simulink model "final_integration"  (R2019b)
settings: Solver=FixedStepDiscrete  StartTime=0.0  StopTime=100  FixedStep=0.1  RelTol=1e-3
undefined symbols (not defined in the file): DiscIntNeverNeededParam, gcbh, rmidispblock, sigbuilder_block
libraries: simulink x2
(part 2 of 2)

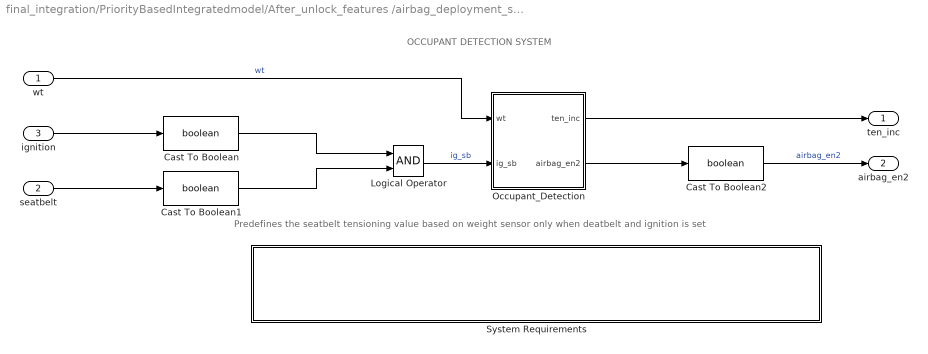
== system final_integration/PriorityBasedIntegratedmodel/After_unlock_features /airbag_deployment_system_main/occuption_detection_system ==
  note: Predefines the seatbelt tensioning value based on weight sensor only when deatbelt and ignition is set
  note: OCCUPANT DETECTION SYSTEM
  wt : Inport
  seatbelt : Inport  Port=2
  ignition : Inport  Port=3
  Cast To Boolean : DataTypeConversion  OutDataTypeStr=boolean
  Cast To Boolean1 : DataTypeConversion  OutDataTypeStr=boolean
  Cast To Boolean2 : DataTypeConversion  OutDataTypeStr=boolean
  Logical Operator : Logic  AllPortsSameDT=off  OutDataTypeStr=boolean
  Occupant_Detection : Stateflow chart  TreatAsAtomicUnit=on
  System Requirements : Subsystem  LoadFcn=rmidispblock('load',gcbh)  mask(System Requirements){id=SystemReq, title=System Requirements}
      mask prompts: title "Block Title"
      mask help: Lists the requirements for the current model.
      mask init:
      | id = 'SystemReq';
      | [w,h] = rmidispblock('display',gcbh);
      settings: CopyFcn=rmidispblock('create',gcbh)  DeleteFcn=rmidispblock('delete',gcbh)  ModelCloseFcn=rmidispblock('close',gcbh)  PreSaveFcn=rmidispblock('close',gcbh)  PostSaveFcn=rmidispblock('open',gcbh)  OpenFcn=rmidispblock('open',gcbh)  MoveFcn=rmidispblock('move',gcbh)
      mask Help: helpview(fullfile(docroot,'slrequirements','helptargets.map'),'systemrequirements')
      mask Display: text(566/2,73-4,rmidispblock('title',gcbh),'horizontalAlignment','center','verticalAlignment','top')
  ten_inc : Outport
  airbag_en2 : Outport  Port=2
  wires:
  Logical Operator/1 -> Occupant_Detection/2(ig_sb)  "ig_sb"
  Cast To Boolean1/1 -> Logical Operator/2
  Cast To Boolean/1 -> Logical Operator/1
  Occupant_Detection/1(ten_inc) -> ten_inc/1
  ignition/1 -> Cast To Boolean/1
  seatbelt/1 -> Cast To Boolean1/1
  Occupant_Detection/2(airbag_en2) -> Cast To Boolean2/1
  Cast To Boolean2/1 -> airbag_en2/1  "airbag_en2"
  wt/1 -> Occupant_Detection/1(wt)  "wt"

== system final_integration/PriorityBasedIntegratedmodel/After_unlock_features /seatbelt_warning_system/System Requirements ==
  Subsystem : Subsystem  mask{label=0, index=1}
      mask init:
      | label = rmidispblock('label',index);
      settings: OpenFcn=rmidispblock('openReq',gcbh);
      mask Display: text(0,0,label,'horizontalAlignment','left','verticalAlignment','bottom')

== system final_integration/PriorityBasedIntegratedmodel/After_unlock_features /suspension_system/System Requirements ==
  Subsystem : Subsystem  mask{label=0, index=1}
      mask init:
      | label = rmidispblock('label',index);
      settings: OpenFcn=rmidispblock('openReq',gcbh);
      mask Display: text(0,0,label,'horizontalAlignment','left','verticalAlignment','bottom')

== system final_integration/PriorityBasedIntegratedmodel/Passive Keyless Entry system/System Requirements/Subsystem ==

== system final_integration/PriorityBasedIntegratedmodel/After_unlock_features /airbag_deployment_system_main/Safe_distance_enable/System Requirements ==
  Subsystem : Subsystem  mask{label=0, index=1}
      mask init:
      | label = rmidispblock('label',index);
      settings: OpenFcn=rmidispblock('openReq',gcbh);
      mask Display: text(0,0,label,'horizontalAlignment','left','verticalAlignment','bottom')

== system final_integration/PriorityBasedIntegratedmodel/After_unlock_features /airbag_deployment_system_main/System Requirements/Subsystem ==

== system final_integration/PriorityBasedIntegratedmodel/After_unlock_features /airbag_deployment_system_main/airbag_decisionsystem/System Requirements ==
  Subsystem : Subsystem  mask{label=0, index=1}
      mask init:
      | label = rmidispblock('label',index);
      settings: OpenFcn=rmidispblock('openReq',gcbh);
      mask Display: text(0,0,label,'horizontalAlignment','left','verticalAlignment','bottom')

== system final_integration/PriorityBasedIntegratedmodel/After_unlock_features /airbag_deployment_system_main/occuption_detection_system/System Requirements ==
  Subsystem : Subsystem  mask{label=0, index=1}
      mask init:
      | label = rmidispblock('label',index);
      settings: OpenFcn=rmidispblock('openReq',gcbh);
      mask Display: text(0,0,label,'horizontalAlignment','left','verticalAlignment','bottom')

== system final_integration/PriorityBasedIntegratedmodel/After_unlock_features /seatbelt_warning_system/System Requirements/Subsystem ==

== system final_integration/PriorityBasedIntegratedmodel/After_unlock_features /suspension_system/System Requirements/Subsystem ==

== system final_integration/PriorityBasedIntegratedmodel/After_unlock_features /airbag_deployment_system_main/Safe_distance_enable/System Requirements/Subsystem ==

== system final_integration/PriorityBasedIntegratedmodel/After_unlock_features /airbag_deployment_system_main/airbag_decisionsystem/System Requirements/Subsystem ==

== system final_integration/PriorityBasedIntegratedmodel/After_unlock_features /airbag_deployment_system_main/occuption_detection_system/System Requirements/Subsystem ==

== stateflow chart final_integration/PriorityBasedIntegratedmodel/After_unlock_features /airbag_deployment_system_main/airbag_decisionsystem/Airbag_Decision ==
  state normalState
    en, du:
    airbagDeploy=0;
    seatTensioner=0;
  state standbyState
    en, du:
    airbagDeploy=0;
    seatTensioner=1;
  state fireState
    en, du:
    airbagDeploy=1;
    seatTensioner=1;
  note: 1) When no Crash(NormalState):Airbag and seatbelt tensioner are not set.
      | 2) When a crash of low or medium level(StandbyState):Seatbelt is tensioned but airbag deployment and steering retraction doesn’t take place.
      | 3) When a crash of high level(StandbyState):Seatbelt is tensioned and airbag deployment and steering retraction is also activated.
  (default) -> normalState
  standbyState -> fireState [order 1] : [vehicle_speed>=22.54]
  normalState -> standbyState : [vehicle_vol>=Vth]
  standbyState -> fireState [order 3] : [12.88<vehicle_speed<22.54]
  fireState -> standbyState : [vehicle_speed<12.88]
  standbyState -> normalState [order 2] : [vehicle_vol<Vth]
  data: Vth local =1; vehicle_speed input; vehicle_vol input; airbagDeploy output; seatTensioner output

== stateflow chart final_integration/PriorityBasedIntegratedmodel/After_unlock_features /airbag_deployment_system_main/occuption_detection_system/Occupant_Detection ==
  state systemOn
    exit:
    airbag_en2=1;
    (default) -> (junction 15) : % tension adjuster
    (junction 15) -> (junction 16) [order 1] : [wt>=75.0 && wt<=100.0]
    (junction 15) -> (junction 17) [order 2]
    (junction 16) -> (junction 24) : {ten_inc=10.0+Tini;}
    (junction 17) -> (junction 18) [order 1] : [wt>=50.0 && wt<=75.0]
    (junction 17) -> (junction 19) [order 2]
    (junction 18) -> (junction 23) : {ten_inc=20.0+Tini;}
    (junction 19) -> (junction 20) [order 1] : [wt>=25.0 && wt<=50.0]
    (junction 19) -> (junction 21) [order 2] : {ten_inc=Tini;}
    (junction 20) -> (junction 22) : {ten_inc=30.0+Tini;}
    (junction 22) -> (junction 21)
    (junction 23) -> (junction 22)
    (junction 24) -> (junction 23)
    (junction 21) -> (junction 25)
  state systemOff
    exit:
    airbag_en2=0;
  note: 1) Ignition and seatbelt is ON,then in order to avoid harsh tensioning of seat belt we read the weight sensor and accordingly set the tensioning percent.
      | 2) Ignition and Seatbelt is OFF,no seatbelt tensioning predefining takes place.
  (default) -> systemOn
  systemOn -> systemOff : [ig_sb==1.0]
  systemOff -> systemOn : [ig_sb==0]
  data: wt input; Tini local =5; ten_inc output; ig_sb input; airbag_en2 output

== stateflow chart final_integration/PriorityBasedIntegratedmodel/After_unlock_features /seatbelt_warning_system/seat_belt_alert_system ==
  state Idle_state
    en:
    seatoccupiedout=0;
    buzzer=0;
    seatbeltout=0;
  note: Input should be either 0 or 1 only
      |
      | There are 4 states:
      | Idle state: Idle means, engine is off, so there is no output
      | Seatoccupied: When passesnger enters the vehicle this state activates and the passenger seated status will be displayed on screen
      | SeatbeltOn: When seat is occupied and the passenger wears seat belt, then this state activates and the seat belt used status will be displayed
      | Buzzer: When seat is occupied nut the belt is not used, buzzer state activates and belt reminder is desplayed on screen
  state Seatoccupied
    en:
    seatoccupiedout=1;
  state Buzzer
    en:
    seatbeltout=0;
    buzzer=1;
    disp('buzzer on');
  state SeatbeltOn
    en:
    seatbeltout=1;
    buzzer=0;
  (default) -> Idle_state
  Idle_state -> Seatoccupied : [seatoccupied==1]
  SeatbeltOn -> Idle_state : [seatoccupied==0]
  Buzzer -> Idle_state [order 1] : [seatoccupied==0]
  Seatoccupied -> Buzzer [order 2] : [seatbelt==0]
  Buzzer -> SeatbeltOn [order 2] : [seatbelt==1]
  Seatoccupied -> SeatbeltOn [order 1] : [seatbelt==1]
  data: seatoccupied input; seatbelt input; seatoccupiedout output; seatbeltout output; buzzer output; c local

== stateflow chart final_integration/PriorityBasedIntegratedmodel/Passive Keyless Entry system/Door_Status_Scenario1 ==
  note: Scenario 1: When user is moving away from the source
  state PassiveENtryScenario1 [group]
    state ScanOff
    state Available
      state Signal
      state SensorWork
        state DoorSensor
          en:
          DoorEntryStatus_S1=0;
          proximity = 100;
          count=0;
          du:
          count = count +1;
          ex:
          count = 101;
        state VehicleSensor
          en:
          DoorEntryStatus_S1=0;
          proximity=750;
          count=101;
          du:
          count=count +1;
          ex:
          count = 751;
        state OutofRange
          en:
          DoorEntryStatus_S1=1;
          disp('Door is Locked');
          disp('--------------------');
          proximity=900;
          count=751;
          du:
          count=count+1;
          ex:
          count = 901;
        (default) -> DoorSensor
        DoorSensor -> VehicleSensor : [count > proximity] {disp('User moving out of Door Proximity');}
        VehicleSensor -> OutofRange : [count > proximity] {disp('User moving out of Vehicle Proximity');
            |                              disp('---------------------------------------');}
      (default) -> Signal
      SensorWork -> Signal : [Input_signal_S1==900]
      Signal -> SensorWork : [Input_signal_S1>0]{disp('Connection of the signal');
          | disp('---------------------------------------');}
    (default) -> ScanOff : {disp('---------------------------------------');
        | disp('User moving away from vehicle');
        | disp('Scanning for Signal Avalabiltiy');
        | disp('----------------------------------------');}
    Available -> ScanOff : [SignalScanInput==0]
    ScanOff -> Available : [SignalScanInput==1]{disp('Signal Available');
        | disp('---------------------------------------');}
  note: %% Vehicle Sensor
      | % When the signal value goes from 100 to 750, the Vehicle state activates
      | % When it reaches the 750 count, the door locks
  note: %% Door Sensor
      | % When the signal value goes from 0 to 100, the Door state activates
      | % When it reaches the 100 count, the still stays the same
  note: %% Door Status
      | % When both the states are active, only then the output status is given.
      | % Otherwise the door remains open
  data: proximity local; count local; Input_signal_S1 input; DoorEntryStatus_S1 output; SignalScanInput input

== stateflow chart final_integration/PriorityBasedIntegratedmodel/Passive Keyless Entry system/Door_Status_Scenario2 ==
  note: Scenario 2: When user is moving towards source
  state PassiveEntryScenario2 [group]
    state ScanOff
    state Available
      state Signal
      state SensorWork
        state OutofRange
          entry:
          DoorEntryStatus_S2=1;
          proximity = 900;
          count=899;
          during:
          count = count -1;
          exit:
          count = 749;
        state VehicleSensor
          entry:
          DoorEntryStatus_S2=1;
          proximity=750;
          count=749;
          during:
          count=count -1;
          exit:
          count = 99;
        state DoorSensor
          entry:
          DoorEntryStatus_S2=0;
          disp('Door is Unocked');
          disp('Ignition sequence allowed');
          disp('-----------------------------------');
          proximity=100;
          count=99;
          during:
          count=count - 1;
          exit:
          count = 1;
        (default) -> OutofRange
        OutofRange -> VehicleSensor : [count==749] {disp('User moving towards Vehicle Proximity');}
        VehicleSensor -> DoorSensor : [count==99] {disp('User moving towards Door Proximity');
            |                      disp('---------------------------------------');}
      (default) -> Signal
      SensorWork -> Signal : [Input_Signal_S2==0]
      Signal -> SensorWork : [Input_Signal_S2 < 1000] {disp('Connection of the signal');
          |                                          disp('---------------------------------------');}
    (default) -> ScanOff : {disp('---------------------------------------');
        | disp('User moving towards the vehicle');
        | disp('Scanning for Signal Avalabiltiy');
        | disp('----------------------------------------');}
    Available -> ScanOff : [SignalScanInput==0]
    ScanOff -> Available : [SignalScanInput==1]{disp('Signal Available');
        | disp('---------------------------------------');}
  note: %% Door Sensor
      | % When the signal value goes from 100 to 0, the Door state activates
      | % When it reaches the 0 count, the door unlocks
  note: %% Vehicle Sensor
      | % When the signal value goes from 750 to 100, the Vehicle state activates
      | % When it reaches the 100 count, the door locks
  note: %% Door Status
      | % When both the states are active, only then the output status is given.
      | % Otherwise the door remains closed
  data: proximity local; count local; Input_Signal_S2 input; DoorEntryStatus_S2 output; SignalScanInput input

== stateflow chart final_integration/PriorityBasedIntegratedmodel/After_unlock_features /suspension_system/tyremonitoring ==
  state Ignition_OFF
    en:
    F_o_v =0;
    R_o_v=0;
    F_i_v =0;
    R_i_v=0;
  note: Igniton is setpoint generator
      | Scenario 1:
      | -> Lower pressure than threshold value inside suspension chamber. This will make the inlet valves to actuate till the threshold value is obtained.
      | Scenario 2:
      | -> Higher pressure than threshold value inside suspension chamber. This will make the outlet valves to actuate till the pressure is dropped to threshold valve.
      | Scenario 3:
      | -> Ideal pressure inside suspension chamber, so no actuation of inlet and outlet valves.
      | Scenario 4:
      | -> Vehicle is accelerating quickly, This will make the rear inlet valves to actuate.
      | Scenario 5:
      | -> Vehicle is de-accelerating quickly, This will make the front inlet valves to actuate.​
  state Ignition_ON
    state City_mode
      (junction 80) -> (junction 82) : {F_i_v=1;R_i_v=1;F_o_v=0;R_o_v=0}
      (junction 88) -> (junction 35) : [IP_press==50 && Acc_ip >30&&Acc_ip<60]
      (junction 25) -> (junction 88) [order 1]
      (junction 21) -> (junction 80) [order 1] : [IP_press<50]
      (junction 82) -> (junction 25)
      (junction 35) -> (junction 36) : {F_i_v=0;R_i_v=0}
      City_mode -> (junction 21) [order 1]
      (junction 21) -> (junction 25) [order 3] : [IP_press==50]
      (junction 25) -> (junction 40) [order 2] : [IP_press==50 && Acc_ip>60]
      (junction 25) -> (junction 90) [order 3]
      (junction 25) -> (junction 24) [order 4]
      (junction 21) -> (junction 84) [order 2] : [IP_press>50]
      (junction 86) -> (junction 25)
      (junction 40) -> (junction 41) : {F_i_v=0;R_i_v=1}
      (junction 90) -> (junction 45) : [IP_press==50 && Acc_ip <30]
      (junction 45) -> (junction 46) : {F_i_v=1;R_i_v=0}
      (junction 84) -> (junction 86) : {F_o_v=1;R_o_v=1;F_i_v=0;R_i_v=0}
      (junction 46) -> (junction 24) : {F_o_v=0;R_o_v=0}
      (junction 92) -> (junction 24)
      (junction 94) -> (junction 24)
      (junction 41) -> (junction 92) : {F_o_v=0;R_o_v=0}
      (junction 36) -> (junction 94) : {F_o_v=0;R_o_v=0}
    state HIghway_mode
      (junction 96) -> (junction 101) : {F_i_v=1;R_i_v=1;F_o_v=0;R_o_v=0}
      (junction 105) -> (junction 55) : [IP_press==100 && Acc_ip >30&&Acc_ip<60]
      (junction 68) -> (junction 105) [order 1]
      (junction 73) -> (junction 96) [order 1] : [IP_press<100]
      (junction 101) -> (junction 68)
      (junction 55) -> (junction 53) : {F_i_v=0;R_i_v=0}
      HIghway_mode -> (junction 73) [order 1]
      (junction 73) -> (junction 68) [order 3] : [IP_press==100]
      (junction 68) -> (junction 63) [order 2] : [IP_press==100 && Acc_ip >60]
      (junction 68) -> (junction 107) [order 3]
      (junction 68) -> (junction 69) [order 4]
      (junction 73) -> (junction 98) [order 2] : [IP_press>100]
      (junction 103) -> (junction 68)
      (junction 63) -> (junction 57) : {F_i_v=0;R_i_v=1}
      (junction 107) -> (junction 60) : [IP_press==100 && Acc_ip<30]
      (junction 60) -> (junction 64) : {F_i_v=1;R_i_v=0}
      (junction 98) -> (junction 103) : {F_o_v=1;R_o_v=1;F_i_v=0;R_i_v=0}
      (junction 64) -> (junction 69) : {F_o_v=0;R_o_v=0}
      (junction 109) -> (junction 69)
      (junction 111) -> (junction 69)
      (junction 57) -> (junction 109) : {F_o_v=0;R_o_v=0}
      (junction 53) -> (junction 111) : {F_o_v=0;R_o_v=0}
    (default) -> City_mode
    HIghway_mode -> City_mode [order 1] : [M_status==0]
    City_mode -> HIghway_mode [order 1] : [M_status==1]
  (default) -> Ignition_OFF
  Ignition_OFF -> Ignition_ON : [Igni_ip ==1]
  Ignition_ON -> Ignition_OFF : [Igni_ip==0]
  data: IP_press input; M_status input; Acc_ip input; Igni_ip input; F_i_v output; R_i_v output; F_o_v output; R_o_v output
